simulink library "Propulsion"  (R2024a)
settings: Solver=VariableStepAuto  StartTime=0.0  StopTime=10.0  RelTol=1e-3
values from neighbouring files (symbols this model uses):
  alfaf_deg = 0    [Initialization.m]    (also in Initialization_alt2.m; Initialization_cg1.m; Initialization_loop.m; Initialization_v2.m)
  nrho = 0.75    [Initialization.m]    (also in Initialization_alt2.m; Initialization_cg1.m; Initialization_loop.m; Initialization_v2.m)
  nv = -1    [Initialization.m]    (also in Initialization_alt2.m; Initialization_cg1.m; Initialization_loop.m; Initialization_v2.m)
  rho_reference_kgpm3 = 0.9569    [Initialization.m]    (also in Initialization_alt2.m; Initialization_cg1.m; Initialization_loop.m = 1.225; Initialization_v2.m)
  Tmax = 300*745.7/V_reference_mps    (= 2743.22501533)    [Initialization.m]    (also in Initialization_alt2.m; Initialization_cg1.m; Initialization_loop.m = 308.3469; Initialization_v2.m)
  V_reference_mps = 81.55    [Initialization.m]    (also in Initialization_alt2.m; Initialization_cg1.m; Initialization_loop.m = velocidade(end); Initialization_v2.m)
  xf_m = 2.02    [Initialization.m]    (also in Initialization_alt2.m; Initialization_cg1.m; Initialization_loop.m; Initialization_v2.m)
  zf_m = 0.1418    [Initialization.m]    (also in Initialization_alt2.m; Initialization_cg1.m; Initialization_loop.m = -0.1418; Initialization_v2.m)
settings Model: Creator=Caê  LastModifiedBy=Caê
settings RTWCC: GPUComputeCapability=3.5

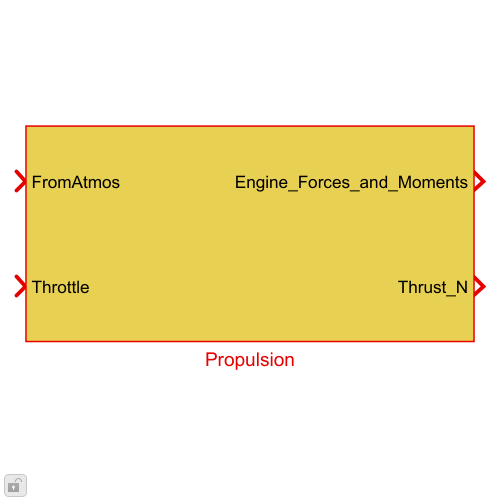
[thumbnail: Simulink's stored preview of the top-level diagram]
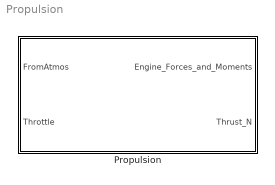
== system Propulsion ==
  Propulsion : Subsystem

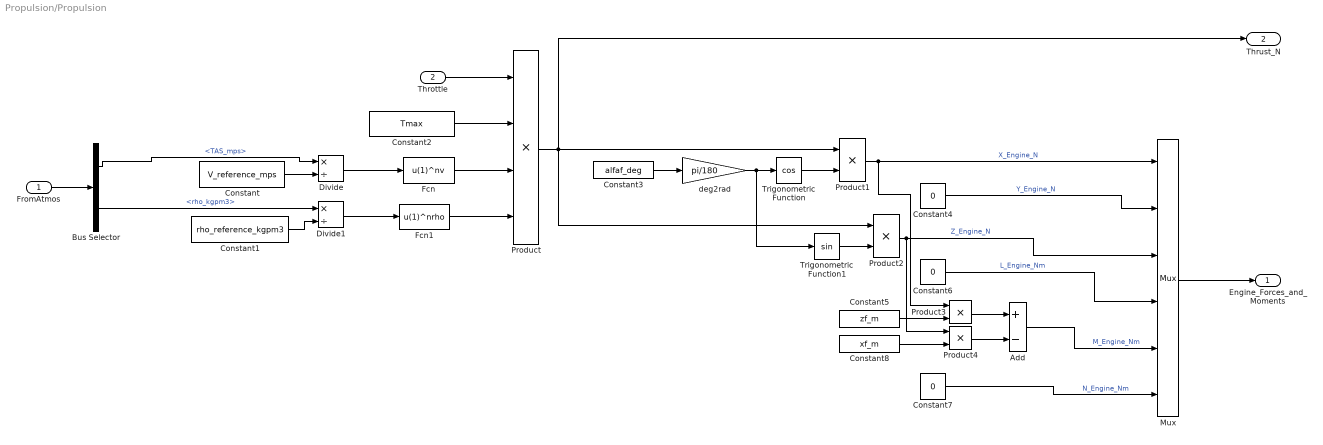
== system Propulsion/Propulsion ==
  FromAtmos : Inport
  Throttle : Inport  Port=2
  Add : Sum  Inputs=+-
  Bus Selector : BusSelector  OutputSignals=TAS_mps,rho_kgpm3
  Constant : Constant  Value=V_reference_mps
  Constant1 : Constant  Value=rho_reference_kgpm3
  Constant2 : Constant  Value=Tmax
  Constant3 : Constant  Value=alfaf_deg
  Constant4 : Constant  Value=0
  Constant5 : Constant  Value=zf_m
  Constant6 : Constant  Value=0
  Constant7 : Constant  Value=0
  Constant8 : Constant  Value=xf_m
  Divide : Product  Inputs=*/
  Divide1 : Product  Inputs=*/
  Fcn : Fcn  Expr=u(1)^nv
  Fcn1 : Fcn  Expr=u(1)^nrho
  Mux : Mux  Inputs=6
  Product : Product  Inputs=4
  Product{1..4} (4 alike) : Product
  Trigonometric Function : Trigonometry  Operator=cos
  Trigonometric Function1 : Trigonometry
  deg2rad : Gain  Gain=pi/180
  Engine_Forces_and_Moments : Outport
  Thrust_N : Outport  Port=2
  wires:
  Mux/1 -> Engine_Forces_and_Moments/1
  Constant2/1 -> Product/2
  Product/1 -> Thrust_N/1, Product2/1, Product1/1
  deg2rad/1 -> Trigonometric Function1/1, Trigonometric Function/1
  Constant3/1 -> deg2rad/1
  Constant6/1 -> Mux/4  "L_Engine_Nm"
  Bus Selector/1 -> Divide/1  "<TAS_mps>"
  Constant7/1 -> Mux/6  "N_Engine_Nm"
  Product4/1 -> Add/2
  FromAtmos/1 -> Bus Selector/1
  Bus Selector/2 -> Divide1/1  "<rho_kgpm3>"
  Fcn/1 -> Product/3
  Throttle/1 -> Product/1
  Product1/1 -> Mux/1, Product3/1  "X_Engine_N"
  Trigonometric Function/1 -> Product1/2
  Divide/1 -> Fcn/1
  Trigonometric Function1/1 -> Product2/2
  Constant8/1 -> Product4/2
  Product2/1 -> Mux/3, Product4/1  "Z_Engine_N"
  Constant/1 -> Divide/2
  Divide1/1 -> Fcn1/1
  Constant5/1 -> Product3/2
  Add/1 -> Mux/5  "M_Engine_Nm"
  Constant4/1 -> Mux/2  "Y_Engine_N"
  Constant1/1 -> Divide1/2
  Fcn1/1 -> Product/4
  Product3/1 -> Add/1
